simulink model "AKident_2015"  (Simulink 8.6)
settings: Solver=ode45  StartTime=0.0  StopTime=tend  MaxStep=0.01  RelTol=1e-3
InitFcn:
  | Tp = 1; %okres próbkowania
  | sigma2v = 0; %wariancja zakłócenia v
  | N = 1001;
  | tend = 1000; %czas symulacji, czy tyle powinien wynosić?
libraries: simulink x1
settings Model: Creator=mgmil  LastModifiedBy=mgmil
settings OptimizationCC: ExpressionDepthLimit=128  InitFltsAndDblsToZero=on
settings DebuggingCC: SaveWithParameterizedLinksMsg=none  SignalResolutionControl=TryResolveAllWithWarning  MultiTaskDSMMsg=warning  MultiTaskCondExecSysMsg=none  FcnCallInpInsideContextMsg=EnableAllAsWarning  AllowSymbolicDim=on  StateNameClashWarn=none
settings SFSimCC: SimUseLocalCustomCode=on
settings RTWCC: RTWUseLocalCustomCode=on
settings GRTTargetCC: TargetFcnLib=ansi_tfl_tmw.mat  GeneratePreprocessorConditionals=Use local settings
settings ConfigComp: CovExternalEMLEnable=on

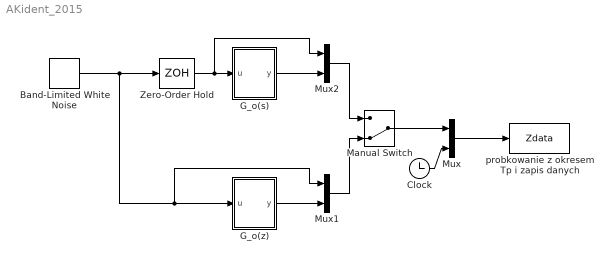
== system AKident_2015 ==
  Band-Limited White Noise : simulink/Sources/Band-Limited White Noise  Cov=[0.5]*Tp  Ts=Tp  seed=[23341]
  Clock : Clock
  G_o(s) : Subsystem
  G_o(z) : Subsystem
  Manual Switch : ManualSwitch  CurrentSetting=0
  Mux : Mux  Inputs=2
  Mux1 : Mux  Inputs=2
  Mux2 : Mux  Inputs=2
  Zero-Order Hold : ZeroOrderHold  SampleTime=Tp
  probkowanie z okresem Tp i zapis danych : ToWorkspace  VariableName=Zdata  SampleTime=Tp
  wires:
  Zero-Order Hold/1 -> G_o(s)/1(u), Mux2/1
  Band-Limited White Noise/1 -> Zero-Order Hold/1, G_o(z)/1(u), Mux1/1
  Mux/1 -> probkowanie z okresem Tp i zapis danych/1
  Manual Switch/1 -> Mux/1
  Clock/1 -> Mux/2
  Mux1/1 -> Manual Switch/2
  Mux2/1 -> Manual Switch/1
  G_o(s)/1(y) -> Mux2/2
  G_o(z)/1(y) -> Mux1/2

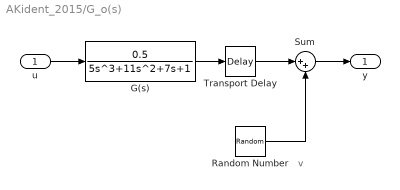
== system AKident_2015/G_o(s) ==
  note: v
  u : Inport
  G(s) : TransferFcn  Numerator=[0.5]  Denominator=[5 11 7 1]
  Random Number : RandomNumber  Variance=sigma2v  Seed=159  SampleTime=Tp*0.1
  Sum : Sum  Inputs=|++
  Transport Delay : TransportDelay  DelayTime=3
  y : Outport
  wires:
  G(s)/1 -> Transport Delay/1
  u/1 -> G(s)/1
  Random Number/1 -> Sum/2
  Sum/1 -> y/1
  Transport Delay/1 -> Sum/1

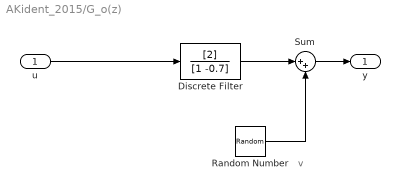
== system AKident_2015/G_o(z) ==
  note: v
  u : Inport
  Discrete Filter : DiscreteFilter  Numerator=[2]  Denominator=[1 -0.7]  SampleTime=Tp
  Random Number : RandomNumber  Variance=sigma2v  Seed=159  SampleTime=Tp
  Sum : Sum  Inputs=|++
  y : Outport
  wires:
  u/1 -> Discrete Filter/1
  Random Number/1 -> Sum/2
  Sum/1 -> y/1
  Discrete Filter/1 -> Sum/1
